simulink model "sim_friction_model"  (R2015b)
settings: Solver=VariableStepAuto  StartTime=0.0  StopTime=10  FixedStep=0.001  RelTol=1e-3
undefined symbols (not defined in the file): lin_sys_A, lin_sys_B, lin_sys_C, lin_sys_D, lin_sys_X
(part 1 of 2)
settings Model: Creator=dave  LastModifiedBy=dave

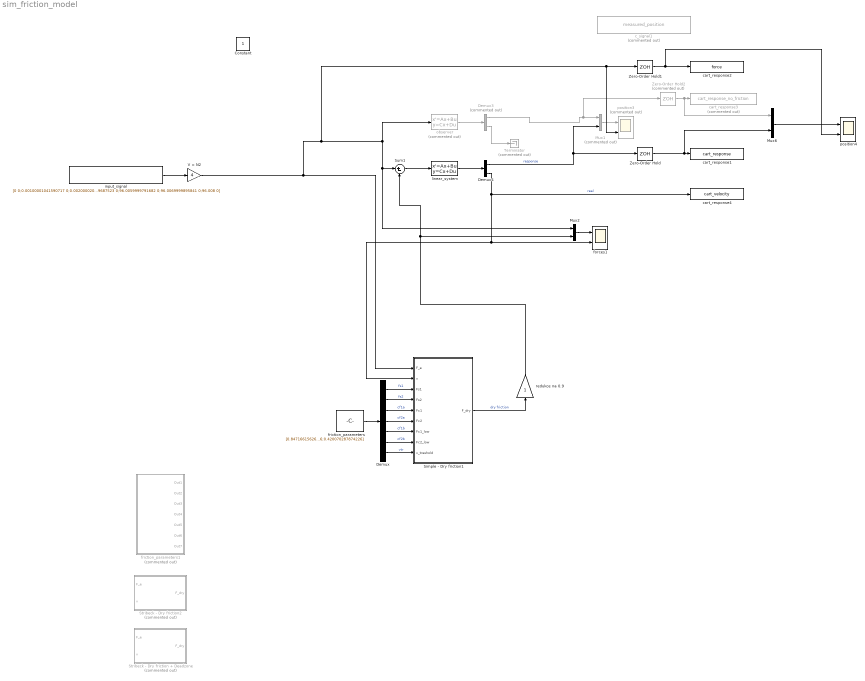
== system sim_friction_model ==
  Demux : Demux  Outputs=7
  Demux3 : Demux  Commented=on  Outputs=2
  Demux4 : Demux  Outputs=2
  Mux1 : Mux  Commented=on  Inputs=2
  Mux2 : Mux  Inputs=2
  Mux6 : Mux  Inputs=2
  Simple - Dry friction1 : MATLAB Function  TreatAsAtomicUnit=on
  Stribeck - Dry friction + Deadzone : MATLAB Function  Commented=on  TreatAsAtomicUnit=on
  Stribeck - Dry friction2 : MATLAB Function  Commented=on  TreatAsAtomicUnit=on
  Sum1 : Sum  Inputs=|+-
  Terminator : Terminator  Commented=on
  V > N2 : Gain  Gain=4
  Zero-Order Hold : ZeroOrderHold  SampleTime=0.001
  Zero-Order Hold1 : ZeroOrderHold  SampleTime=0.001
  Zero-Order Hold2 : ZeroOrderHold  Commented=on  SampleTime=0.001
  c_signal1 : FromWorkspace  Commented=on  VariableName=measured_position  SampleTime=0
  cart_response1 : ToWorkspace  VariableName=cart_response  SaveFormat=Timeseries  SampleTime=-1
  cart_response2 : ToWorkspace  VariableName=force  SaveFormat=Timeseries  SampleTime=-1
  cart_response3 : ToWorkspace  Commented=on  VariableName=cart_response_no_friction  SaveFormat=Timeseries  SampleTime=-1
  cart_response4 : ToWorkspace  VariableName=cart_velocity  SaveFormat=Timeseries  SampleTime=-1
  forces1 : Scope  NumInputPorts=2
  friction_parameters : Constant  Value=[0.847166156268076;0.498614263830718;0.0734317082408059;0.0818507185569055;0.330758018221232;0.253969874939966;0.420070287874226]
  friction_parameters1 : Subsystem  Commented=on
  input_signal : FromWorkspace  VariableName=[0 0;0.00100001041590717 0;0.00200002083181435 0;0.00300003124772152 0;0.00400004166362869 0;0.00500005207953587 0;0.00600006249544304 0;0.00700007291135021 0;0.00800008332725739 0;0.00900009374316456 0;0.0100001041590717 0;0.0110001145749789 0;0.0120001249908861 0;0.0130001354067933 0;0.0140001458227004 0;0.0150001562386076 0;0.0160001666545148 0;0.017000177070422 0;0.0180001874863291 0;0.0190001979022363 0;0.0200002083181435 0;0.0210002187340506 0;0.0220002291499578 0;0.023000239565865 0;0.0240002499817722 0;0.0250002603976793 0;0.0260002708135865 0;0.0270002812294937 0;0.0280002916454009 0;0.029000302061308 0;0.0300003124772152 0;0.0310003228931224 0;0.0320003333090296 0;0.0330003437249367 0;0.0340003541408439 0;0.0350003645567511 0;0.0360003749726582 0;0.0370003853885654 0;0.0380003958044726 0;0.0390004062203798 0;0.0400004166362869 0;0.0410004270521941 0;0.0420004374681013 0;0.0430004478840085 0;0.0440004582999156 0;0.0450004687158228 0;0.04600047913173 0;0.0470004895476372 0;0.0480004999635443 0;0.0490005103794515 0;0.0500005207953587 0;0.0510005312112658 0;0.052000541627173 0;0.0530005520430802 0;0.0540005624589874 0;0.0550005728748945 0;0.0560005832908017 0;0.0570005937067089 0;0.0580006041226161 0;0.0590006145385232 0;0.0600006249544304 0;0.0610006353703376 0;0.0620006457862448 0;0.0630006562021519 0;0.0640006666180591 0;0.0650006770339663 0;0.0660006874498734 0;0.0670006978657806 0;0.0680007082816878 0;0.069000718697595 0;0.0700007291135021 0;0.0710007395294093 0;0.0720007499453165 0;0.0730007603612237 0;0.0740007707771308 0;0.075000781193038 0;0.0760007916089452 0;0.0770008020248524 0;0.0780008124407595 0;0.0790008228566667 0;0.0800008332725739 0;0.0810008436884811 0;0.0820008541043882 0;0.0830008645202954 0;0.0840008749362026 0;0.0850008853521098 0;0.0860008957680169 0;0.0870009061839241 0;0.0880009165998313 0;0.0890009270157384 0;0.0900009374316456 0;0.0910009478475528 0;0.09200095826346 0;0.0930009686793671 0;0.0940009790952743 0;0.0950009895111815 0;0.0960009999270886 0;0.0970010103429958 0;0.098001020758903 0;0.0990010311748102 0;0.100001041590717 0;0.101001052006625 0;0.102001062422532 0;0.103001072838439 0;0.104001083254346 0;0.105001093670253 0;0.10600110408616 0;0.107001114502068 0;0.108001124917975 0;0.109001135333882 0;0.110001145749789 0;0.111001156165696 0;0.112001166581603 0;0.113001176997511 0;0.114001187413418 0;0.115001197829325 0;0.116001208245232 0;0.117001218661139 0;0.118001229077046 0;0.119001239492954 0;0.120001249908861 0;0.121001260324768 0;0.122001270740675 0;0.123001281156582 0;0.12400129157249 0;0.125001301988397 0;0.126001312404304 0;0.127001322820211 0;0.128001333236118 0;0.129001343652025 0;0.130001354067933 0;0.13100136448384 0;0.132001374899747 0;0.133001385315654 0;0.134001395731561 0;0.135001406147468 0;0.136001416563376 0;0.137001426979283 0;0.13800143739519 0;0.139001447811097 0;0.140001458227004 0;0.141001468642911 0;0.142001479058819 0;0.143001489474726 0;0.144001499890633 0;0.14500151030654 0;0.146001520722447 0;0.147001531138355 0;0.148001541554262 0;0.149001551970169 0;0.150001562386076 0;0.151001572801983 0;0.15200158321789 0;0.153001593633798 0;0.154001604049705 0;0.155001614465612 0;0.156001624881519 0;0.157001635297426 0;0.158001645713333 0;0.159001656129241 0;0.160001666545148 0;0.161001676961055 0;0.162001687376962 0;0.163001697792869 0;0.164001708208776 0;0.165001718624684 0;0.166001729040591 0;0.167001739456498 0;0.168001749872405 0;0.169001760288312 0;0.17000177070422 0;0.171001781120127 0;0.172001791536034 0;0.173001801951941 0;0.174001812367848 0;0.175001822783755 0;0.176001833199663 0;0.17700184361557 0;0.178001854031477 0;0.179001864447384 0;0.180001874863291 0;0.181001885279198 0;0.182001895695106 0;0.183001906111013 0;0.18400191652692 0;0.185001926942827 0;0.186001937358734 0;0.187001947774641 0;0.188001958190549 0;0.189001968606456 0;0.190001979022363 0;0.19100198943827 0;0.192001999854177 0;0.193002010270084 0;0.194002020685992 0;0.195002031101899 0 ...(+1815299 chars)]  SampleTime=0
  linear_system : StateSpace  A=[0 1;0 -2.6]  B=[0;0.37037037037037]  C=[1 0;0 1]  D=[0;0]  X0=[0 0]
  observer : StateSpace  Commented=on  A=lin_sys_A  B=lin_sys_B  C=lin_sys_C  D=lin_sys_D  X0=lin_sys_X
  position3 : Scope  Commented=on  NumInputPorts=2
  position4 : Scope  NumInputPorts=2
  redukce na 0.9 : Gain
  Constant : Constant  IOType=siggen
  wires:
  Sum1/1 -> linear_system/1
  observer/1 -> Demux3/1
  linear_system/1 -> Demux4/1
  Demux4/2 -> forces1/2, Simple - Dry friction1/2(v), cart_response4/1  "real"
  Mux2/1 -> forces1/1
  Simple - Dry friction1/1(F_dry) -> redukce na 0.9/1  "dry friction"
  Demux4/1 -> Mux1/2, Zero-Order Hold/1  "response"
  Demux3/2 -> Terminator/1
  Zero-Order Hold1/1 -> position4/2, cart_response2/1
  Demux3/1 -> Zero-Order Hold2/1, Mux1/1
  Mux1/1 -> position3/1
  Zero-Order Hold2/1 -> Mux6/1, cart_response3/1
  redukce na 0.9/1 -> Mux2/2, Sum1/2
  Mux6/1 -> position4/1
  input_signal/1 -> V > N2/1
  Zero-Order Hold/1 -> Mux6/2, cart_response1/1
  V > N2/1 -> Simple - Dry friction1/1(F_e), position3/2, Zero-Order Hold1/1, observer/1, Mux2/1, Sum1/1
  Demux/1 -> Simple - Dry friction1/3(Fs1)  "fs1"
  Demux/2 -> Simple - Dry friction1/4(Fs2)  "fs2"
  Demux/3 -> Simple - Dry friction1/5(Fc1)  "cf1a"
  Demux/4 -> Simple - Dry friction1/6(Fc2)  "cf2a"
  Demux/5 -> Simple - Dry friction1/7(Fc1_low)  "cf1b"
  Demux/6 -> Simple - Dry friction1/8(Fc2_low)  "cf2b"
  Demux/7 -> Simple - Dry friction1/9(v_treshold)  "vtr"
  friction_parameters/1 -> Demux/1
